simulink model "PV_System"  (R2025a)
settings: Solver=VariableStepAuto  StartTime=0.0  StopTime=10  RelTol=1e-3
PreLoadFcn:
  | % === Load 1-D LUT (25 °C irradiance sweep) ===
  | if exist('pmpp_25C_from_plot.mat','file')
  |     S1 = load('pmpp_25C_from_plot.mat');
  |     assignin('base','G_vec',     S1.G_vec);
  |     assignin('base','Pmpp_vals', S1.Pmpp_vals);
  | end
  | 
  | % === Load 2-D LUT (G,T table) ===
  | if exist('pmpp_G_T_table.mat','file')
  |     S2 = load('pmpp_G_T_table.mat');
  |     assignin('base','G_grid',    S2.G_grid);
  |     assignin('base','T_grid',    S2.T_grid);
  |     assignin('base','Pmpp_table',S2.Pmpp_table);
  | end
values from neighbouring files (symbols this model uses):
  G_grid = Sg.G_vec(:).'    [LUT_Merge.m]    (also in pmpp_G_T_table.mat = [200 300 400 500 600 700 800 900 1000])
  G_vec = G_vec(1:n)    [FigDataExtractor.m]    (also in pmpp_25C_from_plot.mat = [200 300 400 500 600 700 800 900 1000])
  Pmpp_table = scale_T(:) * Pmpp_G_at_25(:).'    [LUT_Merge.m]    (also in pmpp_G_T_table.mat = [10.2413826915 9.34693440985 8.3912575092 7.37988388849 15.6)
  Pmpp_vals = Pmpp_vals(1:n)    [FigDataExtractor.m]    (also in pmpp_25C_from_plot.mat = [9.34693440985 14.266894956 19.2347849953 24.2295623967 29.2)
  T_grid = T_grid(1:n)    [FidDataExtractorTemp.m]    (also in LUT_Merge.m = St.T_grid(:).'; pmpp_1000_vs_T.mat = [0 25 50 75]; pmpp_G_T_table.mat = [0 25 50 75])
undefined symbols (not defined in the file or in its folder): Acid, DiscIntNeverNeededParam, Lead
libraries: spsSeriesRLCBranchLib x9, spsCurrentMeasurementLib x2, spsDiodeLib x2, spsVoltageMeasurementLib x2, SignalEditorBlockLib x2, spsIGBTDiodeLib x1, spsBatteryLib x1, spsMosfetLib x1, spsPVArrayLib x1, slpidlib x1, spsPWMGeneratorDCDCLib x1, sps_lib x1
settings Model: Creator=bista  LastModifiedBy=joshg

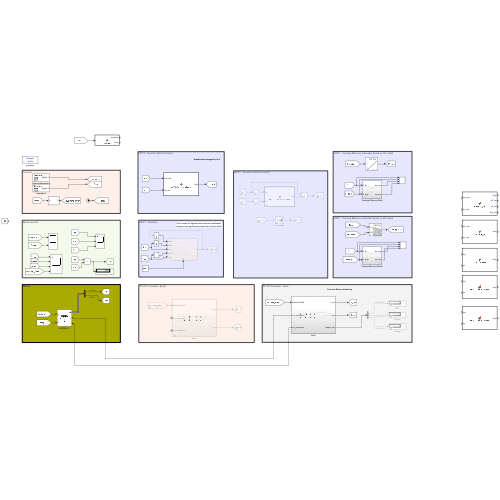
[thumbnail: Simulink's stored preview of the top-level diagram]
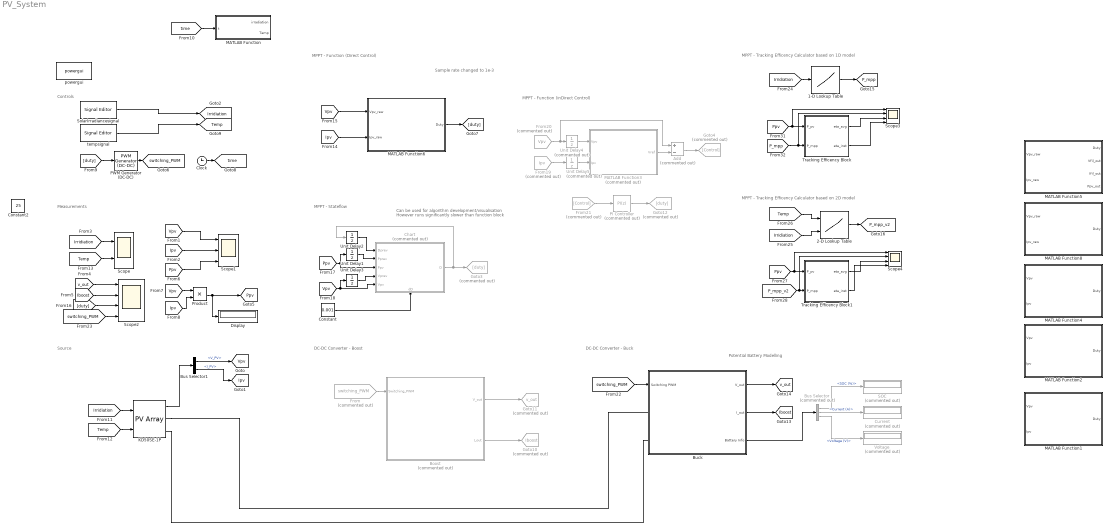
== system PV_System ==
  note: Can be used for algorithm development/visualisation
      | However runs significantly slower than function block
  note: Measurements
  note: Source
  note: Controls
  note: MPPT - Stateflow
  note: MPPT - Function (Direct Control)
  note: DC-DC Converter - Boost
  note: Potential Battery Modelling
  note: MPPT - Function (inDirect Control)
  note: DC-DC Converter - Buck
  note: Sample rate changed to 1e-3
  note: MPPT - Tracking Efficency Calculator based on 1D model
  note: MPPT - Tracking Efficency Calculator based on 2D model
  1-D Lookup Table : Lookup_n-D  NumberOfTableDimensions=1  BreakpointsForDimension1=G_vec  Table=Pmpp_vals  InternalRulePriority=Speed  RndMeth=Simplest
  2-D Lookup Table : Lookup_n-D  BreakpointsForDimension1=T_grid  BreakpointsForDimension2=G_grid  Table=Pmpp_table  InternalRulePriority=Speed  RndMeth=Simplest
      settings: InputPortMap=u0,u1
  Add : Sum  Commented=on  Inputs=+-
  Boost : Subsystem  Commented=on
  Buck : Subsystem
  Bus Selector : BusSelector  Commented=on  OutputSignals=SOC (%),Current (A),Voltage (V)
  Bus Selector1 : BusSelector  OutputSignals=V_PV,I_PV
  Chart : Stateflow chart  Commented=on  TreatAsAtomicUnit=on
      settings: PortSchema="{\"entries\":[{\"content\":{\"sides\":[{\"content\":{\"connectorIds\":[\"In1\",\"In2\",\"In3\",\"In5\",\"In6\"]},\"type\":\"ConnectorPlacement.EquallySpacedRectSide\",\"uuid\":\"d9c2b273-da21-4eaa-8b85-3980967242cf\"},{\"content\":{\"connectorIds\":[\"Out1\"],\"side\":\"RIGHT\"},\"type\":\"ConnectorPlacement.EquallySpacedRectSide\",\"uuid\":\"5d89ac01-9659-48cd-85be-cd83dc39a4f4\"},{\"content\":{\"side\":\"TOP\"},\"type\":\"ConnectorPlacement.EquallySpacedRectSide\",\"uuid\":\"137de6a3-6666-4d5d-9076-10c036d2112d\"},{\"content\":{\"connectorIds\":[\"In4\"],\"side\":\"BOTTOM\"},\"type\":\"ConnectorPlacement.EquallySpacedRectSide\",\"uuid\":\"26e6fe93-d823-44bf-a4e3-6882e06f529a\"}]},\"type\":\"ConnectorPlacement.EquallySpacedConnector\",\"uuid\":\"9c29b58e-f51c-4562-afea-24f99672fb48\"}],\"packageUris\":[\"http://schema.mathworks.com/mf0/Connector/R2020b\"],\"version\":\"1.0\"}"
  Clock : Clock
  Constant : Constant  Value=0.001
  Constant2 : Constant  Value=25
  Current : Display  Commented=on
  Display : Display
  From : From  Commented=on  GotoTag=switching_PWM  TagVisibility=global
  From19 : From  Commented=on  GotoTag=Ipv  TagVisibility=global
  From20 : From  Commented=on  GotoTag=Vpv  TagVisibility=global
  From21 : From  Commented=on  GotoTag=Control
  Goto10 : Goto  Commented=on  GotoTag=Iboost  TagVisibility=global
  Goto11 : Goto  Commented=on  GotoTag=v_out  TagVisibility=global
  Goto12 : Goto  Commented=on  GotoTag=duty
  Goto3 : Goto  Commented=on  GotoTag=duty
  Goto4 : Goto  Commented=on  GotoTag=Control
  KD50SE-1P : spsPVArrayLib/PV Array  Npar=1  Nser=1  PlotType=array @ 1000 W/m2 & specified temperatures  S_vec=[ 1000 900 800 700 600 500 400 300 200]  Temp_C_vec=[ 0 25 50 75]  ModuleName=User-defined  PlotWhenSelected=off  Pm=50.12  Ncell=36  Voc=19.9  Isc=3  Vm=17.9  Im=2.80  beta_Voc_pc=-0.1  alpha_Isc_pc=0.102  beta_Voc=-0.0199  alpha_Isc=0.00306  IL=3.0001  I0=2.8355e-10  nI=1.0003  Rsh=179.0004  Rs=0.23334  RobustModel=off  RobustCellTemperature=313.3991  BAL=on  Tc=1e-6  Tfilter=5e-5
  MATLAB Function : MATLAB Function  TreatAsAtomicUnit=on
  MATLAB Function1 : MATLAB Function  TreatAsAtomicUnit=on
  MATLAB Function2 : MATLAB Function  TreatAsAtomicUnit=on
  MATLAB Function3 : MATLAB Function  Commented=on  TreatAsAtomicUnit=on
  MATLAB Function4 : MATLAB Function  TreatAsAtomicUnit=on
  MATLAB Function5 : MATLAB Function  TreatAsAtomicUnit=on
  MATLAB Function6 : MATLAB Function  TreatAsAtomicUnit=on
  MATLAB Function8 : MATLAB Function  TreatAsAtomicUnit=on
  PI Controller : slpidlib/PID Controller  Commented=on  Controller=PI  Form=Parallel  TimeDomain=Discrete-time  UseExternalTs=off  SampleTime=500e-6  IntegratorMethod=Forward Euler  FilterMethod=Forward Euler  ControllerParametersSource=internal  P=0.05  I=5  UseKiTs=off  D=0  UseExternalDerivativeSource=off  N=100  UseFilter=on  TunerSelectOption=Transfer Function Based (PID Tuner App)  InitialConditionSource=internal  InitialConditionForIntegrator=0.2  InitialConditionForFilter=0  DifferentiatorICPrevScaledInput=0  ExternalReset=none  TrackingMode=off  Kt=1  LimitOutput=on  SatLimitsSource=internal  UpperSaturationLimit=0.95  LowerSaturationLimit=0.1  LinearizeAsGain=on  AntiWindupMode=none  Kb=1  LimitIntegrator=off  UpperIntegratorSaturationLimit=inf  LowerIntegratorSaturationLimit=-inf  POutMin=[]  POutMax=[]  IOutMin=[]  IOutMax=[]  DOutMin=[]  DOutMax=[]  NOutMin=[]  NOutMax=[]  SumOutMin=[]  SumOutMax=[]  SaturationOutMin=[]  SaturationOutMax=[]  PParamMin=[]  PParamMax=[]  IParamMin=[]  IParamMax=[]  DParamMin=[]  DParamMax=[]  NParamMin=[]  NParamMax=[]  KbParamMin=[]  KbParamMax=[]  KtParamMin=[]  KtParamMax=[]  KbOutMin=[]  KbOutMax=[]  KtOutMin=[]  KtOutMax=[]  IntegratorOutMin=[]  IntegratorOutMax=[]  FilterOutMin=[]  FilterOutMax=[]  SumI1OutMin=[]  SumI1OutMax=[]  SumI2OutMin=[]  SumI2OutMax=[]  SumI3OutMin=[]  SumI3OutMax=[]  SumI4OutMin=[]  SumI4OutMax=[]  SumDOutMin=[]  SumDOutMax=[]  DifferentiatorOutMin=[]  DifferentiatorOutMax=[]  FilterDiffOutCoefMin=[]  FilterDiffOutCoefMax=[]  ReciprocalOutMin=[]  ReciprocalOutMax=[]  SumDenOutMin=[]  SumDenOutMax=[]  SumNumOutMin=[]  SumNumOutMax=[]  DivideOutMin=[]  DivideOutMax=[]  UdiffTsProdOutMin=[]  UdiffTsProdOutMax=[]  NTsProdOutMin=[]  NTsProdOutMax=[]  UintegralTsProdOutMin=[]  UintegralTsProdOutMax=[]  UngainTsProdOutMin=[]  UngainTsProdOutMax=[]  ClampingZeroOutDataTypeStr=Inherit: Inherit via back propagation  ClampingZeroOutMin=[]  ClampingZeroOutMax=[]  FilterDenConstantOutDataTypeStr=Inherit: Inherit via back propagation  FilterDenConstantOutMin=[]  FilterDenConstantOutMax=[]  PCopyOutDataTypeStr=Inherit: Inherit via back propagation  PCopyOutMin=[]  PCopyOutMax=[]  NCopyOutDataTypeStr=Inherit: Inherit via back propagation  NCopyOutMin=[]  NCopyOutMax=[]  IntegratorContinuousStateAttributes=''  IntegratorStateMustResolveToSignalObject=off  IntegratorRTWStateStorageClass=Auto  FilterContinuousStateAttributes=''  FilterStateMustResolveToSignalObject=off  FilterRTWStateStorageClass=Auto  ParallelPVariant=InternalParameters  IdealPVariant=Disabled  IVariant=InternalParameters  DVariant=Disabled  IntegratorVariant=Discrete  SatVariant=Enabled  AWVariant=Passthrough  PCopyVariant=Disabled  TRVariant=Disabled  FdbkBlocksVariant=Forward  IdealPFdbkVariant=Disabled  SatFdbkVariant=Disabled  DerivativeFilterVariant=Disabled  NVariant=Disabled  NCopyVariant=Disabled_SignalSpec  FilterICVariant=Disabled  IntegratorICVariant=InternalICs  ExternalResetVariant=Disabled  TRSumVariant=Passthrough  SumFdbkVariant=Disabled  SumVariant=Sum_PI  TsampFilterVariant=InternalTs  TsampNgainVariant=Passthrough  TsampIntegralVariant=Disabled_SignalSpec  ExternalSaturationOutDataTypeStr=Inherit: Same as second input  DerivativeSourceVariant=Disabled  PreIntVariant=InternalPreInt
  PWM Generator (DC-DC) : spsPWMGeneratorDCDCLib/PWM Generator (DC-DC)  Fsw=50000  Ts=1e-6
  Product : Product
  SOC : Display  Commented=on
  Scope : Scope  NumInputPorts=2
      settings: ActiveDisplayYMinimum=-96.874999999999972  ActiveDisplayYMaximum=1121.875
  Scope1 : Scope  NumInputPorts=3
      settings: ActiveDisplayYMinimum=-2.4970921279632927  ActiveDisplayYMaximum=22.522282131535079
  Scope2 : Scope  NumInputPorts=4
      settings: ActiveDisplayYMinimum=-1.2198511385562294  ActiveDisplayYMaximum=10.97866024748039  DataLoggingVariableName=ScopeData2
  Scope3 : Scope  NumInputPorts=4
      settings: Title=Tracking Efficency  ActiveDisplayYMinimum=-7.4186615263985933  ActiveDisplayYMaximum=50.082217748189  DataLoggingVariableName=ScopeData3
  Scope4 : Scope  NumInputPorts=4
      settings: Title=Tracking Efficency  ActiveDisplayYMinimum=0.67954306868631664  ActiveDisplayYMaximum=2.7213997425614194  DataLoggingVariableName=ScopeData4
  SolarIrradiancesignal : SignalEditorBlockLib/Signal Editor  FileName=SolarIrradiance_50step.mat  ActiveScenario=Scenario  ActiveSignal=Signal 1  IsBus=off  OutputBusObjectStr=Bus: BusObject  SampleTime=0  ZeroCross=off  OutputAfterFinalValue=Setting to zero  Unit=inherit  PreserveSignalName=on  ApplySigPropsToAllScenarios=on  ApplySigPropsToAllSignals=off  SignalPropertySource=Dialog parameters
  Tracking Efficency Block : Subsystem
  Tracking Efficency Block1 : Subsystem
  Unit Delay1 : UnitDelay  SampleTime=-1  HasFrameUpgradeWarning=on
  Unit Delay2 : UnitDelay  SampleTime=-1  HasFrameUpgradeWarning=on
  Unit Delay3 : UnitDelay  SampleTime=-1  HasFrameUpgradeWarning=on
  Unit Delay4 : UnitDelay  Commented=on  SampleTime=1e-4  HasFrameUpgradeWarning=on
  Unit Delay5 : UnitDelay  Commented=on  SampleTime=1e-4  HasFrameUpgradeWarning=on
  Voltage : Display  Commented=on
  powergui : sps_lib/powergui  Priority=1  SimulationMode=Discrete  SampleTime=1e-6  frequency=60  Iterations=50  frequencyindice=0  Pbase=100e6  ErrMax=1e-4  UnitsV=kV  UnitsW=MW  buscounter=0  FunctionMessages=off  echomessages=off  EnableUseOfTLC=off  CurrentSourceSwitches=off  DisableSnubberDevices=off  DisableRonSwitches=off  DisableVfSwitches=off  DisplayEquations=off  AutomaticDiscreteSolvers=off  SolverType=Tustin/Backward Euler (TBE)  Interpol=off  ExternalGateDelay=off  methode=off  Ts=100  x0status=blocks  SPID=on  SwTol=0  HookPort=off  NonlinearTolerance=1e-4  nMaxIteration=100  ContinueOnMaxIteration=off  RestoreLinks=warning  ResistiveCurrentMeasurement=off  Frange=[0:2:500]  Ylog=off  Xlog=on  ShowGrid=off  save=off  variable=ZData  structure=0  ZoomFFT=off  StartTime=0.0  cycles=1  DisplayStyle=1  fundamental=60  FreqAxis=off  MaxFrequency=1000  frequencyindicesteady=1  RmsSteady=1  display=off
  tempsignal : SignalEditorBlockLib/Signal Editor  FileName=SolarTemp_25step.mat  ActiveScenario=Scenario  ActiveSignal=Signal 1  IsBus=off  OutputBusObjectStr=Bus: BusObject  SampleTime=0  ZeroCross=off  OutputAfterFinalValue=Setting to zero  Unit=inherit  PreserveSignalName=on  ApplySigPropsToAllScenarios=on  ApplySigPropsToAllSignals=off  SignalPropertySource=Dialog parameters
  tag scope: Iboost=global, Ipv=global, Irridiation=global, P_mpp=global, P_mpp_v2=global, Ppv=global, Temp=global, Vpv=global, switching_PWM=global, time=global, v_out=global
  wires:
  Product/1 -> Display/1, [Ppv]
  [Vpv] -> Product/1
  [Ipv] -> Product/2
  KD50SE-1P/1 -> Bus Selector1/1
  Clock/1 -> [time]
  [Irridiation] -> KD50SE-1P/1
  [Temp] -> KD50SE-1P/2
  [Irridiation] -> Scope/1
  [Temp] -> Scope/2
  [Ipv] -> Scope1/2
  [Ppv] -> Scope1/3
  [time] -> MATLAB Function/1(t)
  PWM Generator (DC-DC)/1 -> [switching_PWM]
  [duty] -> PWM Generator (DC-DC)/1
  [Vpv] -> Scope1/1
  [v_out] -> Scope2/1
  [Iboost] -> Scope2/2
  [duty] -> Scope2/3
  From/1 -> Boost/1(Switching_PWM)
  Boost/1(V_out) -> Goto11/1
  Boost/2(I_out) -> Goto10/1
  Chart/1(D) -> Unit Delay2/1, Goto3/1
  Unit Delay2/1 -> Chart/1(Dprev)
  [Ppv] -> Chart/3(Ppv), Unit Delay1/1
  Unit Delay1/1 -> Chart/2(Pprev)
  [Vpv] -> Chart/6(Vpv), Unit Delay3/1
  Unit Delay3/1 -> Chart/5(Vprev)
  Constant/1 -> Chart/4(dD)
  Buck/3(Battery Info) -> Bus Selector/1
  Bus Selector/2 -> Current/1  "<Current (A)>"
  Bus Selector/1 -> SOC/1  "<SOC (%)>"
  Bus Selector/3 -> Voltage/1  "<Voltage (V)>"
  From20/1 -> Add/1, Unit Delay4/1
  Unit Delay4/1 -> MATLAB Function3/1(Vpv)
  Unit Delay5/1 -> MATLAB Function3/2(Ipv)
  From19/1 -> Unit Delay5/1
  MATLAB Function3/1(Vref) -> Add/2
  Add/1 -> Goto4/1
  From21/1 -> PI Controller/1
  PI Controller/1 -> Goto12/1
  Buck/1(V_out) -> [v_out]
  Buck/2(I_out) -> [Iboost]
  [switching_PWM] -> Buck/1(Switching PWM)
  Bus Selector1/1 -> [Vpv]  "<V_PV>"
  Bus Selector1/2 -> [Ipv]  "<I_PV>"
  [switching_PWM] -> Scope2/4
  [Ipv] -> MATLAB Function6/2(Ipv_raw)
  SolarIrradiancesignal/1 -> [Irridiation]
  tempsignal/1 -> [Temp]
  [Vpv] -> MATLAB Function6/1(Vpv_raw)
  MATLAB Function6/1(Duty) -> [duty]
  [Irridiation] -> 1-D Lookup Table/1
  1-D Lookup Table/1 -> [P_mpp]
  [Ppv] -> Scope3/1, Tracking Efficency Block/1(P_pv)
  [P_mpp] -> Scope3/2, Tracking Efficency Block/2(P_mpp)
  Tracking Efficency Block/2(eta_inst) -> Scope3/4
  Tracking Efficency Block/1(eta_avg) -> Scope3/3
  [Temp] -> 2-D Lookup Table/1
  [Irridiation] -> 2-D Lookup Table/2
  2-D Lookup Table/1 -> [P_mpp_v2]
  Tracking Efficency Block1/2(eta_inst) -> Scope4/4
  [Ppv] -> Scope4/1, Tracking Efficency Block1/1(P_pv)
  [P_mpp_v2] -> Scope4/2, Tracking Efficency Block1/2(P_mpp)
  Tracking Efficency Block1/1(eta_avg) -> Scope4/3
  connections:
  KD50SE-1P/RConn1 -- Buck/LConn1
  KD50SE-1P/RConn2 -- Buck/LConn2

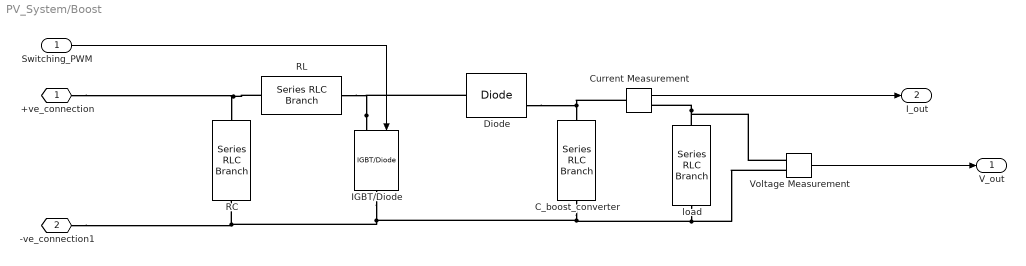
== system PV_System/Boost ==
  Switching_PWM : Inport
  C_boost_converter : spsSeriesRLCBranchLib/Series RLC Branch  LConnTagsString=__new0  RConnTagsString=__new0  BranchType=RC  Resistance=1e-4  Inductance=1e-3  SetiL0=off  InitialCurrent=0  Capacitance=3300e-6  Setx0=off  InitialVoltage=0  Measurements=None
  Current Measurement : spsCurrentMeasurementLib/Current Measurement  PhasorSimulation=off  OutputType=Complex  PSBequivalent=0
  Diode : spsDiodeLib/Diode  Ron=0.001  Lon=0  Vf=0.8  IC=0  UseSnubber=0  Rs=500  Cs=250e-9  Measurements=on
  IGBT/Diode : spsIGBTDiodeLib/IGBT//Diode  Ron=1e-3  Rs=1e5  Cs=inf  Measurements=off
  RC : spsSeriesRLCBranchLib/Series RLC Branch  LConnTagsString=__new0  RConnTagsString=__new0  BranchType=RC  Resistance=1e-4  Inductance=1e-3  SetiL0=off  InitialCurrent=0  Capacitance=100e-6  Setx0=off  InitialVoltage=0  Measurements=None
  RL : spsSeriesRLCBranchLib/Series RLC Branch  LConnTagsString=__new0  RConnTagsString=__new0  BranchType=RL  Resistance=0.1  Inductance=47e-6  SetiL0=off  InitialCurrent=0  Capacitance=100e-6  Setx0=off  InitialVoltage=0  Measurements=None
  Voltage Measurement : spsVoltageMeasurementLib/Voltage Measurement  PhasorSimulation=off  OutputType=Complex  PSBequivalent=0
  load : spsSeriesRLCBranchLib/Series RLC Branch  LConnTagsString=__new0  RConnTagsString=__new0  BranchType=R  Resistance=2.88  Inductance=5e-3  SetiL0=off  InitialCurrent=0  Capacitance=100e-6  Setx0=off  InitialVoltage=0  Measurements=None
  +ve_connection : PMIOPort  Side=Left
  -ve_connection1 : PMIOPort  Port=2  Side=Left
  V_out : Outport
  I_out : Outport  Port=2
  wires:
  Current Measurement/1 -> I_out/1
  Voltage Measurement/1 -> V_out/1
  Switching_PWM/1 -> IGBT/Diode/1
  connections:
  load/LConn1 -- Current Measurement/RConn1 -- Voltage Measurement/LConn1
  C_boost_converter/LConn1 -- Diode/RConn1 -- Current Measurement/LConn1
  load/RConn1 -- Voltage Measurement/LConn2 -- C_boost_converter/RConn1 -- IGBT/Diode/RConn1 -- RC/RConn1 -- -ve_connection1/RConn1
  RL/RConn1 -- +ve_connection/RConn1 -- RC/LConn1
  IGBT/Diode/LConn1 -- RL/LConn1 -- Diode/LConn1

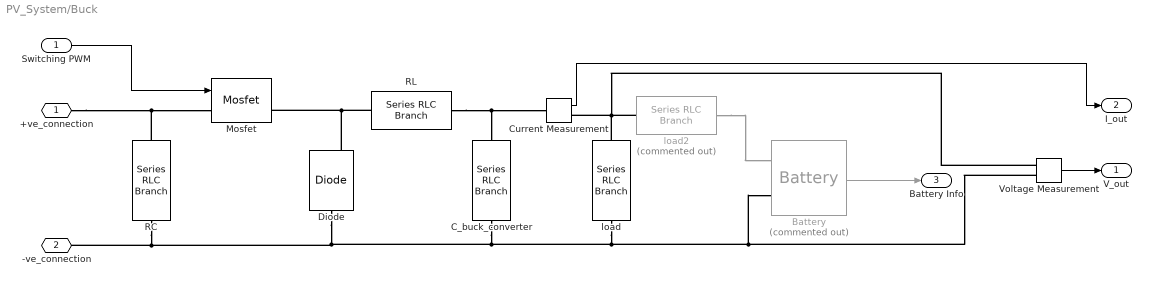
== system PV_System/Buck ==
  Switching PWM : Inport
  Battery : spsBatteryLib/Battery  Commented=on  BatType=Lead-Acid  NomV=12  NomQ=100  SOC=45  Batt_Tr=1  PresetModel=on  MaxQ=104.1667  MinV=9  FullV=13.0658  Dis_rate=20  R=0.0012  Normal_OP=31.0278  expZone="[12.2171     0.333333]"
  C_buck_converter : spsSeriesRLCBranchLib/Series RLC Branch  LConnTagsString=__new0  RConnTagsString=__new0  BranchType=RC  Resistance=1e-4  Inductance=1e-3  SetiL0=off  InitialCurrent=0  Capacitance=470e-6  Setx0=off  InitialVoltage=0  Measurements=None
      settings: AttributesFormatString=%<Capacitance>
  Current Measurement : spsCurrentMeasurementLib/Current Measurement  PhasorSimulation=off  OutputType=Complex  PSBequivalent=0
  Diode : spsDiodeLib/Diode  Ron=0.001  Lon=0  Vf=0.8  IC=0  UseSnubber=0  Rs=500  Cs=250e-9  Measurements=on
  Mosfet : spsMosfetLib/Mosfet  Ron=0.1  Lon=0  Rd=0.01  Vfd=0  IC=0  Rs=1e5  Cs=inf  Measurements=on
  RC : spsSeriesRLCBranchLib/Series RLC Branch  LConnTagsString=__new0  RConnTagsString=__new0  BranchType=RC  Resistance=1e-4  Inductance=1e-3  SetiL0=off  InitialCurrent=0  Capacitance=330e-6  Setx0=off  InitialVoltage=0  Measurements=None
      settings: AttributesFormatString=%<Capacitance>
  RL : spsSeriesRLCBranchLib/Series RLC Branch  LConnTagsString=__new0  RConnTagsString=__new0  BranchType=RL  Resistance=0.1  Inductance=47e-6  SetiL0=off  InitialCurrent=0  Capacitance=100e-6  Setx0=off  InitialVoltage=0  Measurements=None
      settings: AttributesFormatString=%<Inductance>
  Voltage Measurement : spsVoltageMeasurementLib/Voltage Measurement  PhasorSimulation=off  OutputType=Complex  PSBequivalent=0
  load : spsSeriesRLCBranchLib/Series RLC Branch  LConnTagsString=__new0  RConnTagsString=__new0  BranchType=R  Resistance=2.88  Inductance=5e-3  SetiL0=off  InitialCurrent=0  Capacitance=100e-6  Setx0=off  InitialVoltage=0  Measurements=None
  load2 : spsSeriesRLCBranchLib/Series RLC Branch  Commented=on  LConnTagsString=__new0  RConnTagsString=__new0  BranchType=R  Resistance=0.1  Inductance=5e-3  SetiL0=off  InitialCurrent=0  Capacitance=100e-6  Setx0=off  InitialVoltage=0  Measurements=None
  +ve_connection : PMIOPort  Side=Left
  -ve_connection : PMIOPort  Port=2  Side=Left
  V_out : Outport
  I_out : Outport  Port=2
  Battery Info : Outport  Port=3
  wires:
  Switching PWM/1 -> Mosfet/1
  Voltage Measurement/1 -> V_out/1
  Current Measurement/1 -> I_out/1
  Battery/1 -> Battery Info/1
  connections:
  load/LConn1 -- Voltage Measurement/LConn1 -- load2/RConn1 -- Current Measurement/RConn1
  RL/RConn1 -- Diode/RConn1 -- Mosfet/RConn1
  Diode/LConn1 -- Voltage Measurement/LConn2 -- Battery/LConn2 -- load/RConn1 -- C_buck_converter/RConn1 -- RC/RConn1 -- -ve_connection/RConn1
  +ve_connection/RConn1 -- RC/LConn1 -- Mosfet/LConn1
  RL/LConn1 -- Current Measurement/LConn1 -- C_buck_converter/LConn1
  load2/LConn1 -- Battery/LConn1

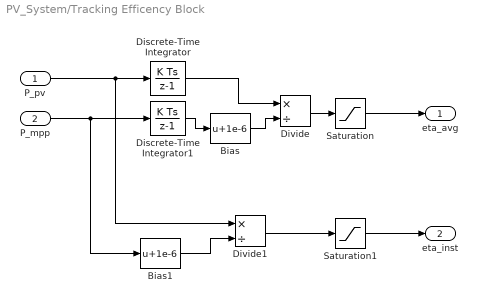
== system PV_System/Tracking Efficency Block ==
  P_pv : Inport
  P_mpp : Inport  Port=2
  Bias : Bias  Bias=1e-6  SaturateOnIntegerOverflow=off
  Bias1 : Bias  Bias=1e-6  SaturateOnIntegerOverflow=off
  Discrete-Time Integrator : DiscreteIntegrator  SampleTime=1e-3  UpperSaturationLimit=1  LowerSaturationLimit=0  ICPrevOutput=DiscIntNeverNeededParam  ICPrevScaledInput=DiscIntNeverNeededParam
  Discrete-Time Integrator1 : DiscreteIntegrator  SampleTime=1e-3  UpperSaturationLimit=1  LowerSaturationLimit=0  ICPrevOutput=DiscIntNeverNeededParam  ICPrevScaledInput=DiscIntNeverNeededParam
  Divide : Product  Inputs=*/
  Divide1 : Product  Inputs=*/
  Saturation : Saturate  UpperLimit=1  LowerLimit=0
  Saturation1 : Saturate  UpperLimit=1  LowerLimit=0
  eta_avg : Outport
  eta_inst : Outport  Port=2
  wires:
  P_pv/1 -> Divide1/1, Discrete-Time Integrator/1
  Discrete-Time Integrator/1 -> Divide/1
  Bias1/1 -> Divide1/2
  P_mpp/1 -> Bias1/1, Discrete-Time Integrator1/1
  Saturation1/1 -> eta_inst/1
  Divide/1 -> Saturation/1
  Discrete-Time Integrator1/1 -> Bias/1
  Bias/1 -> Divide/2
  Saturation/1 -> eta_avg/1
  Divide1/1 -> Saturation1/1

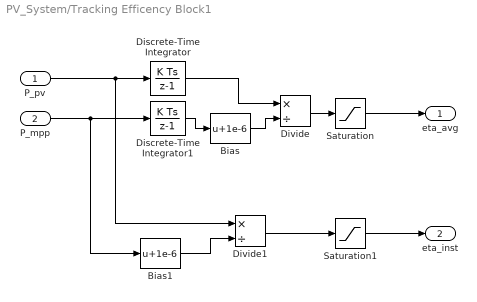
== system PV_System/Tracking Efficency Block1 ==
  P_pv : Inport
  P_mpp : Inport  Port=2
  Bias : Bias  Bias=1e-6  SaturateOnIntegerOverflow=off
  Bias1 : Bias  Bias=1e-6  SaturateOnIntegerOverflow=off
  Discrete-Time Integrator : DiscreteIntegrator  SampleTime=1e-3  UpperSaturationLimit=1  LowerSaturationLimit=0  ICPrevOutput=DiscIntNeverNeededParam  ICPrevScaledInput=DiscIntNeverNeededParam
  Discrete-Time Integrator1 : DiscreteIntegrator  SampleTime=1e-3  UpperSaturationLimit=1  LowerSaturationLimit=0  ICPrevOutput=DiscIntNeverNeededParam  ICPrevScaledInput=DiscIntNeverNeededParam
  Divide : Product  Inputs=*/
  Divide1 : Product  Inputs=*/
  Saturation : Saturate  UpperLimit=1  LowerLimit=0
  Saturation1 : Saturate  UpperLimit=1  LowerLimit=0
  eta_avg : Outport
  eta_inst : Outport  Port=2
  wires:
  P_pv/1 -> Divide1/1, Discrete-Time Integrator/1
  Discrete-Time Integrator/1 -> Divide/1
  Bias1/1 -> Divide1/2
  P_mpp/1 -> Bias1/1, Discrete-Time Integrator1/1
  Saturation1/1 -> eta_inst/1
  Divide/1 -> Saturation/1
  Discrete-Time Integrator1/1 -> Bias/1
  Bias/1 -> Divide/2
  Saturation/1 -> eta_avg/1
  Divide1/1 -> Saturation1/1

== matlab function PV_System/MATLAB Function6 ==
  settings: updateMethod=DISCRETE  sampleTime=1e-3
  data: Duty output; Vpv_raw input; Ipv_raw input
function Duty = ASSATA_currentZone(Vpv_raw, Ipv_raw)
% ASSTA (Adjustable Step Size Theta) with Current-Zone Clamp (Alg. 4 hybrid)
% - Keeps your simple atan(dP/dV) and dθ/dV proxy
% - Adds a learned I_MPP estimate and ±% zone that freezes duty near MPP
% - Removes early-return on tiny dV (uses surrogate dV instead)

% ---------- Your original tunables ----------
C        = 0.003;     % deadband on M
Z        = 0.02;      % dθ/dV threshold
SF       = 0.10;      % step scale
Dmin     = 0.00;
Dmax     = 0.95;
Dinit    = 0.50;

% ---------- Robustness ----------
EPS_DV   = 1e-4;      % floor for |dV|
EPS_TH   = 1e-3;      % |θ|≈0 band
EPS_M    = 1e-5;      % tiny M floor

% ---------- Duty slew ----------
Ts_ctrl   = 1e-3;     % controller tick (s)
SLEW_RATE = 5.0;      % max duty change per second
DSTEPMAX  = SLEW_RATE * Ts_ctrl;

% ---------- Measurement filtering ----------
ALPHA     = 0.20;     % EMA on V/I

% ---------- Current-zone (Alg. 4) ----------
IZONE_PCT = 0.03;     % Band around I_MPP estimate
ALPHA_IMP = 0.05;     % I_MPP estimate smoothing

% ---------- Persistent states ----------
persistent Vold Iold Pold Dold Vfil Ifil init_done ...
           Imp_hat     % running estimate of I_MPP

if isempty(init_done)
    Vfil      = Vpv_raw;
    Ifil      = Ipv_raw;
    Vold      = Vfil;
    Iold      = Ifil;
    Pold      = Vfil * Ifil;
    Dold      = Dinit;
    Imp_hat   = max(Ifil, 0);   % seed I_MPP estimate with first current
    init_done = true;
end

% ---------- EMA filtering ----------
Vfil = (1 - ALPHA) * Vfil + ALPHA * Vpv_raw;
Ifil = (1 - ALPHA) * Ifil + ALPHA * Ipv_raw;

% ---------- Deltas ----------
Ppv  = Vfil * Ifil;
dVpv = Vfil - Vold;
dIpv = Ifil - Iold;
dPpv = Ppv  - Pold;

% Surrogate dV (avoid freeze/div-by-zero)
dV_eff = dVpv;
if abs(dV_eff) < EPS_DV
    dV_eff = sign(dV_eff) * EPS_DV;
end

% ---------- ASSTA core metrics ----------
M        = abs(dPpv + dIpv * dVpv);  if M < EPS_M, M = 0; end
ratio    = dPpv / dV_eff;
theta    = atan(ratio);              % simple θ
dtheta_dv = 1 / (1 + ratio^2);       % book's proxy equation

% ---------- Near-MPP detector ----------
near_mpp = (abs(theta) < EPS_TH) && (dtheta_dv > Z);

% Update I_MPP estimate only when we're confidently near MPP
if near_mpp
    Imp_hat = (1 - ALPHA_IMP) * Imp_hat + ALPHA_IMP * max(Ifil, 0);
end

% ---------- Current-zone clamp ----------
I_low  = Imp_hat * (1 - IZONE_PCT);
I_high = Imp_hat * (1 + IZONE_PCT);
in_zone = (Ifil >= I_low) && (Ifil <= I_high);

% ---------- Decision logic ----------
Duty = Dold;

if in_zone
    % Inside learned MPP current band → freeze duty (zero ripple at MPP)
    Duty = Dold;
elseif M >= C
    % Outside the band = normal ASSTA step
    delta = SF * M;
    if (abs(theta) < EPS_TH) && (dtheta_dv > Z)
        Duty = Dold;  % extra guard if gate triggers
    else
        if theta > 0
            Duty = Dold - delta;
        else
            Duty = Dold + delta;
        end
    end
else
    % Tiny change → hold
    Duty = Dold;
end

% ---------- Slew and clamps ----------
Duty = max(min(Duty, Dold + DSTEPMAX), Dold - DSTEPMAX);
Duty = min(max(Duty, Dmin), Dmax);

% ---------- Store ----------
Dold = Duty;
Vold = Vfil;
Iold = Ifil;
Pold = Ppv;

end

== matlab function PV_System/MATLAB Function8 ==
  settings: updateMethod=DISCRETE  sampleTime=1e-3
  data: Duty output; Vpv_raw input; Ipv_raw input
function Duty = ASSATA_fil(Vpv_raw, Ipv_raw)
% ASSTA (Adjustable Step Size Theta Approach)
% With measurement filtering to reduce noise in Vpv and Ipv

% --- Tunables ---
C        = 0.003;     % Deadband threshold for M
Z        = 0.02;      % Threshold for dtheta/dV
SF       = 0.10;      % Scaling factor (0.1–0.3 for stability)
Dmin     = 0.00;      % Minimum duty cycle
Dmax     = 0.95;      % Maximum duty cycle
Dinit    = 0.50;      % Initial duty cycle

% --- Robustness knobs ---
EPS_DV   = 1e-4;      % Treat |dV| < EPS_DV as zero (avoid div by 0)
EPS_TH   = 1e-3;      % "theta ≈ 0" band (radians)
EPS_M    = 1e-5;      % Treat very small M as zero
DSTEPMAX = 1e-3;    % Maximum duty change per iteration

% --- Filtering knob ---
ALPHA    = 0.2;       % IIR smoothing factor (0<ALPHA<=1)

% --- Persistent states ---
persistent Vold Iold Pold Dold Vfil Ifil init_done

% Initialize persistent variables on first call
if isempty(init_done)
    Vfil      = Vpv_raw;
    Ifil      = Ipv_raw;
    Vold      = Vfil;
    Iold      = Ifil;
    Pold      = Vfil * Ifil;
    Dold      = Dinit;
    init_done = true;
end

% --- Apply IIR filtering to raw signals ---
Vfil = (1 - ALPHA) * Vfil + ALPHA * Vpv_raw;
Ifil = (1 - ALPHA) * Ifil + ALPHA * Ipv_raw;

% --- Compute PV power and deltas (using filtered signals) ---
Ppv  = Vfil * Ifil;
dVpv = Vfil - Vold;
dIpv = Ifil - Iold;
dPpv = Ppv  - Pold;

% --- Guard against very small dV (unstable slope calc) ---
if abs(dVpv) < EPS_DV
    Duty = Dold;
    Vold = Vfil;
    Iold = Ifil;
    Pold = Ppv;
    Dold = Duty;
    return
end

% --- Adjustable step size (eq. 4.17 from book) ---
M = abs(dPpv + dIpv * dVpv);
if M < EPS_M
    M = 0;
end

% --- Theta and derivative of theta (eq. 4.15) ---
ratio     = dPpv / dVpv;
theta     = atan(ratio);
dtheta_dv = 1 / (1 + ratio^2);

% --- Decision logic with safe default (hold duty) ---
Duty = Dold;

if M >= C
    if (abs(theta) < EPS_TH) && (dtheta_dv > Z)
        % At or near MPP, hold duty
        Duty = Dold;
    else
        % Otherwise adjust duty by scaled step size
        delta = SF * M;
        if theta > 0
            Duty = Dold - delta;   % Move one way
        else
            Duty = Dold + delta;   % Move the other way
        end
    end
else
    % If change in power is too small, hold duty
    Duty = Dold;
end

% --- Limit maximum per-iteration duty step ---
Duty = max(min(Duty, Dold + DSTEPMAX), Dold - DSTEPMAX);

% --- Clamp to absolute duty cycle limits ---
Duty = min(max(Duty, Dmin), Dmax);

% --- Store states for next iteration ---
Dold = Duty;
Vold = Vfil;
Iold = Ifil;
Pold = Ppv;

end

== matlab function PV_System/MATLAB Function1 ==
  settings: updateMethod=DISCRETE  sampleTime=1e-3
  data: Duty output; Vpv input; Ipv input
function Duty = MPPT_PandO_Buck(Vpv, Ipv) 
Dmax = 0.95;
Dmin = 0;
Dinit = 0.5;
deltaD = 125e-6;

persistent Vold Pold Dold;

datatype = 'double';


%initialization for 1st run
if isempty(Vold)
    Vold = 0;
    Pold = 0;
    Dold = Dinit;
end

Ppv = Vpv*Ipv;
dVpv = Vpv - Vold;
dPpv = Ppv - Pold;


if(dPpv ~= 0)
    if(dPpv < 0)
          if(dVpv < 0)
               Duty = Dold - deltaD;
          else
               Duty = Dold + deltaD;
          end
    else
          if(dVpv < 0)
               Duty = Dold + deltaD;
          else
               Duty = Dold - deltaD;
          end
    end
else
    Duty = Dold;
end

if Duty >= Dmax || Duty < Dmin
    Duty = Dold;
end

Dold = Duty;
Vold = Vpv;
Pold = Ppv;

== matlab function PV_System/MATLAB Function ==
  data: irradiation output; t input; Temp output
function [irradiation, Temp] = weather(t)

    Temp = 25;   % constant temperature

    % Parameters
    G_start   = 1000;   % W/m^2 initial irradiance
    G_end     = 500;    % W/m^2 final irradiance
    t_start   = 5;      % time when transition begins
    t_ramp    = 2;      % duration of transition (seconds)

    if t < t_start
        irradiation = G_start;
    elseif t < t_start + t_ramp
        % Linear ramp from G_start to G_end
        frac = (t - t_start) / t_ramp;
        irradiation = G_start + frac * (G_end - G_start);
    else
        irradiation = G_end;
    end

end

== matlab function PV_System/MATLAB Function2 ==
  settings: updateMethod=DISCRETE  sampleTime=1e-3
  data: Duty output; Vpv input; Ipv input
function Duty = MPPT_PandO_Buck(Vpv, Ipv) 
Dmax = 0.95;
Dmin = 0;
Dinit = 0.5;
deltaD = 125e-6;

persistent Vold Pold Dold;

datatype = 'double';


%initialization for 1st run
if isempty(Vold)
    Vold = 0;
    Pold = 0;
    Dold = Dinit;
end

Ppv = Vpv*Ipv;
dVpv = Vpv - Vold;
dPpv = Ppv - Pold;


if(dPpv ~= 0)
    if(dPpv < 0)
          if(dVpv < 0)
               Duty = Dold - deltaD;
          else
               Duty = Dold + deltaD;
          end
    else
          if(dVpv < 0)
               Duty = Dold + deltaD;
          else
               Duty = Dold - deltaD;
          end
    end
else
    Duty = Dold;
end

if Duty >= Dmax || Duty < Dmin
    Duty = Dold;
end

Dold = Duty;
Vold = Vpv;
Pold = Ppv;

== stateflow chart PV_System/Chart ==
  state calculate
    dP=Ppv-Pprev;
    dV=Vpv-Vprev
  state dP_bigger
  state dP_smaller
  state IncreaseD
    D=Dprev+dD;
  state Return
    D=max(0.1, min(0.9, D))
  state DecreaseD
    D=Dprev-dD;
  Return -> calculate
  (default) -> calculate
  calculate -> dP_bigger [order 1] : [dP>0]
  dP_bigger -> IncreaseD [order 2] : [dV<0]
  dP_bigger -> DecreaseD [order 1] : [dV>0]
  calculate -> dP_smaller [order 2] : [dP<0]
  dP_smaller -> IncreaseD [order 2] : [dV>0]
  IncreaseD -> Return
  dP_smaller -> DecreaseD [order 1] : [dV<0]
  DecreaseD -> Return
  data: Dprev input; Pprev input; Ppv input; dD input; dP local; D output =0.5; Vprev input; Vpv input; dV local

== matlab function PV_System/MATLAB Function3 ==
  data: Vref output; Vpv input; Ipv input
function Vref = MPPT_PandO_inDirect(Vpv, Ipv)

Vrefmax = 18.5;
Vrefmin = 13;
Vrefinit = 17.9;
deltaVref = 0.05;
persistent Vold Pold Vrefold

dataType = 'double'

%initialization for 1st run
if isempty(Vold)
    Vold = 0;
    Pold = 0;
    Vrefold = Vrefinit;
end

 Ppv = Vpv*Ipv;
 dPpv = Ppv - Pold;
 dVpv = Vpv - Vold;

 if(dPpv ~= 0)
     if(dPpv<0)
           if(dVpv<0)
                Vref = Vrefold + deltaVref;
           else
                Vref = Vrefold - deltaVref;
           end
     else
           if(dVpv<0)
                Vref = Vrefold - deltaVref;
           else
                Vref = Vrefold + deltaVref;
           end
     end
 else
     Vref = Vrefold;
 end

 if Vref >= Vrefmax || Vref <= Vrefmin
     Vref = Vrefold;
 end

 Vold = Vpv;
 Pold = Ppv;
 Vrefold = Vref;
end

== matlab function PV_System/MATLAB Function4 ==
  data: Duty output; Vpv input; Ipv input
function Duty = ASSATA_nofil(Vpv, Ipv)
% ASSTA (Adjustable Step Size Theta Approach) — buck/boost compatible

% --- Tunables ---
C        = 0.003;    % deadband for M
Z        = 0.02;     % threshold for dtheta/dV
SF       = 0.10;     % scaling factor (0.1–0.3)
Dmin     = 0.00;
Dmax     = 0.95;
Dinit    = 0.50;

% NEW: robustness knobs
EPS_DV   = 1e-4;     % treat |dV| < EPS_DV as zero
EPS_TH   = 1e-3;     % "theta ≈ 0" band (rad)
EPS_M    = 1e-5;     % tiny M treated as zero
DSTEPMAX = 125e-6;   % max duty change per iteration

persistent Vold Iold Pold Dold
if isempty(Vold); Vold = Vpv; Iold = Ipv; Pold = Vpv*Ipv; Dold = Dinit; end

% Deltas between samples
Ppv  = Vpv*Ipv;
dVpv = Vpv - Vold;
dIpv = Ipv - Iold;
dPpv = Ppv - Pold;

% Guard small dV
if abs(dVpv) < EPS_DV
    % no reliable slope; hold duty & update stores
    Duty = Dold;
    Vold = Vpv; Iold = Ipv; Pold = Ppv; Dold = Duty;
    return
end

% Adjustable step size (book eq)
M = abs(dPpv + dIpv*dVpv);
if M < EPS_M
    M = 0;
end

% θ and dθ/dV (with guard)
ratio      = dPpv / dVpv;
theta      = atan(ratio);
dtheta_dv  = 1 / (1 + ratio^2);   % as per book’s simplification

% Decision logic with bands
Duty = Dold;

if M >= C
    if (abs(theta) < EPS_TH) && (dtheta_dv > Z)
        % stay
        Duty = Dold;
    else
        delta = SF * M;
        % direction by sign(theta)
        if theta > 0
            Duty = Dold - delta;
        else
            Duty = Dold + delta;
        end
    end
else
    Duty = Dold;
end

% Limit per-tick slew
Duty = max(min(Duty, Dold + DSTEPMAX), Dold - DSTEPMAX);

% Clamp to absolute limits
Duty = min(max(Duty, Dmin), Dmax);

% Store state
Dold = Duty; Vold = Vpv; Iold = Ipv; Pold = Ppv;
end

== matlab function PV_System/MATLAB Function5 ==
  settings: updateMethod=DISCRETE  sampleTime=1e-3
  data: Duty output; Vpv_raw input; Ipv_raw input; Vfil_out output; Ifil_out output; Ppv_out output
function [Duty, Vfil_out, Ifil_out, Ppv_out] = ASSATA_v2(Vpv_raw, Ipv_raw)
% ASSTA (Adjustable Step Size Theta Approach)
% Tuned for buck converter (signs fixed).
% Includes IIR filtering, numerical dθ/dV, and rate-based duty limiting.
% Now exports filtered V, I, and P for debugging/plotting.

% ---------- Tunables ----------
C         = 0.003;    % deadband on M (book default)
Z         = 0.02;     % dθ/dV threshold near-MPP (book default)
SF        = 0.20;     % step scale (gentler for stability, book 0.1–0.3)
Dmin      = 0.00;     
Dmax      = 0.95;     
Dinit     = 0.50;     

% Controller timing and rate limits
Ts_ctrl   = 1e-3;     % controller sample time (s)
SLEW_RATE = 5.0;      % max duty change per second (faster response)
DSTEPMAX  = SLEW_RATE * Ts_ctrl;  % per-tick duty cap

% Filtering
ALPHA     = 0.3;      % EMA smoothing factor (smoother, less ripple)

% Robustness epsilons
EPS_DV    = 1e-4;     % floor for |dV|
EPS_TH    = 1e-3;     % |θ| ~ 0 band (rad)
EPS_M     = 1e-6;     % floor on M

% ---------- Persistent states ----------
persistent Vold Iold Pold Dold Vfil Ifil init_done theta_old Vold_for_dtheta
if isempty(init_done)
    Vfil = Vpv_raw;
    Ifil = Ipv_raw;
    Vold = Vfil;
    Iold = Ifil;
    Pold = Vfil*Ifil;
    Dold = Dinit;
    theta_old = 0;
    Vold_for_dtheta = Vold;
    init_done = true;
end

% ---------- IIR filtering ----------
Vfil = (1 - ALPHA) * Vfil + ALPHA * Vpv_raw;
Ifil = (1 - ALPHA) * Ifil + ALPHA * Ipv_raw;

% ---------- PV power and deltas ----------
Ppv  = Vfil * Ifil;
dVpv = Vfil - Vold;
dIpv = Ifil - Iold;
dPpv = Ppv  - Pold;

% Use surrogate dV when very small
if abs(dVpv) < EPS_DV
    dV_eff = sign(dVpv) * EPS_DV;
else
    dV_eff = dVpv;
end

% Adaptive step magnitude
M = abs(dPpv + dIpv * dVpv);
if M < EPS_M, M = 0; end

% θ and numerical dθ/dV
ratio     = dPpv / dV_eff;
theta     = atan(ratio);
dtheta_dv = (theta - theta_old) / max(abs(Vfil - Vold_for_dtheta), EPS_DV);

% ---------- Decision logic ----------
Duty = Dold;  % default hold

if M >= C
    if (abs(theta) < EPS_TH) && (dtheta_dv > Z)
        % near MPP → hold
        Duty = Dold;
    else
        % adjust duty by scaled step size
        delta = SF * M;
        if theta > 0
            Duty = Dold - delta;   % static sign convention for buck
        else
            Duty = Dold + delta;
        end
    end
end

% ---------- Limit duty step and clamp ----------
Duty = max(min(Duty, Dold + DSTEPMAX), Dold - DSTEPMAX);
Duty = min(max(Duty, Dmin), Dmax);

% ---------- Store states ----------
Dold            = Duty;
Vold            = Vfil;
Iold            = Ifil;
Pold            = Ppv;
theta_old       = theta;
Vold_for_dtheta = Vfil;

% ---------- Export filtered signals ----------
Vfil_out = Vfil;
Ifil_out = Ifil;
Ppv_out  = Ppv;

end
